simulink model "alignment_bending_procedure_n_4"  (R2018b)
settings: Solver=VariableStepAuto  StartTime=0.0  StopTime=3  RelTol=1e-3
values from neighbouring files (symbols this model uses):
  base_size = [0.2 0.3 1.5]    [robot_setup.m]    (also in robot_setup_bis.m)
  beam_length = 1.14    [robot_setup.m]    (also in robot_setup_bis.m)
  beam_radius = 0.032    [robot_setup.m]    (also in robot_setup_bis.m)
  beam_state_wf_des = fixture_keypoints(fixture_height, fixture_y, n_keypoints)    [robot_setup.m]    (also in robot_setup_bis.m)
  fixture_height = 1.5    [robot_setup.m]    (also in robot_setup_bis.m)
  fixture_x = 0.8    [robot_setup.m]    (also in robot_setup_bis.m)
  J = fscanf(fileID, '    [jacobian_mean_std.m]    (also in robot_setup.m = J_array{i-n_start+1}; robot_setup_bis.m = J_array{i-n_start+1})
  n_keypoints = i    [robot_setup.m]    (also in robot_setup_bis.m)
  robot_frame_x = 0.15    [robot_setup.m]    (also in robot_setup_bis.m)
  T = 0.005    [robot_setup.m]    (also in robot_setup_bis.m; sim_robot_control_error.m)
  wf_T_rf_left = [R_left, xyz_left'; 0 0 0 1]    [robot_setup.m]    (also in robot_setup_bis.m)
  wf_T_rf_right = [R_right, xyz_right'; 0 0 0 1]    [robot_setup.m]    (also in robot_setup_bis.m)
  xyz_0_rf_left = xyz_0_rf_left(1:3)    [robot_setup.m]    (also in robot_setup_bis.m)
  xyz_0_rf_right = xyz_0_rf_right(1:3)    [robot_setup.m]    (also in robot_setup_bis.m)
undefined symbols (not defined in the file or in its folder): beam_wall, beam_width, Extr_Data_Box, Levenberg, Marquardt, X, Y, Z
libraries: sm_lib x329, nesl_utility x49, sm_flex_body_lib x12, robotcorelib x4, simulink x2, robotmaniplib x2
(part 8 of 8)

== system alignment_bending_procedure_n_4/KUKA LWR right/KUKA_iiwa 1 /iiwa_link_7 ==
  Inertia : sm_lib/Body Elements/Inertia  InertiaType=Custom  Mass=3.129  MassUnits=kg  CenterOfMass=[0, 0, 0]  CenterOfMassUnits=m  MomentsOfInertia=[0.01464, 0.01465, 0.002872]  MomentsOfInertiaUnits=kg*m^2  ProductsOfInertia=[0, 0, 0.0005912]  ProductsOfInertiaUnits=kg*m^2  GraphicType=None  MarkerShape=Inertia  MarkerSize=20  GraphicVisPropType=SimpleVisualProperties  GraphicDiffuseColor=[0.5 0.5 0.5]  GraphicSpecularColor=[0.5 0.5 0.5 1.0]  GraphicAmbientColor=[0.15 0.15 0.15 1.0]  GraphicEmissiveColor=[0.0 0.0 0.0 1.0]  GraphicShininess=75  GraphicOpacity=1.0
  InertiaOriginTransform : sm_lib/Frames and Transforms/Rigid Transform  TranslationMethod=Cartesian  TranslationStandardOffset=0  TranslationLengthUnit=m  TranslationStandardAxis=+Z  TranslationCartesianOffset=[0, 0, 0.02]  TranslationROffset=0  TranslationROffsetUnits=m  TranslationZOffset=0  TranslationZOffsetUnits=m  TranslationThetaOffset=0  TranslationThetaOffsetUnits=deg  RotationMethod=RotationSequence  RotationAngleUnits=deg  RotationStandardAxis=+Z  RotationAngle=0.0  RotationArbitraryAxis=[0 0 1]  FollAlignAxisA=+X  BaseAlignAxisA=+Y  FollAlignAxisB=+Y  BaseAlignAxisB=+Z  RotationSequenceAxes=BaseAxes  RotationSequence=XYZ  RotationSequenceAngles=[0, 0, 0]  RotationSequenceAnglesUnits=rad  RotationMatrix=[1 0 0; 0 1 0; 0 0 1]
  ReferenceFrame : sm_lib/Frames and Transforms/Reference Frame
  Visual : sm_lib/Body Elements/Solid  InertiaType=Custom  Mass=0  MassUnits=kg  CenterOfMass=[0, 0, 0]  CenterOfMassUnits=m  MomentsOfInertia=[0, 0, 0]  MomentsOfInertiaUnits=kg*m^2  ProductsOfInertia=[0, 0, 0]  ProductsOfInertiaUnits=kg*m^2  BasedOnType=Density  Density=1000  DensityUnits=kg/m^3  DoExposeReferenceFrame=on  SerializedFrames=<Frames/>  GraphicType=FromGeometry  MarkerShape=Sphere  MarkerSize=10  GraphicVisPropType=SimpleVisualProperties  GraphicDiffuseColor=[0.4, 0.4, 0.4]  GraphicSpecularColor=[0.5 0.5 0.5 1.0]  GraphicAmbientColor=[0.15 0.15 0.15 1.0]  GraphicEmissiveColor=[0.0 0.0 0.0 1.0]  GraphicShininess=75  GraphicOpacity=1  GeometryShape=FromFile  RectangleSize=[1 1]  RectangleSizeUnits=m  BrickDimensions=[1 1 1]  BrickDimensionUnits=m  CylinderRadius=1  CylinderRadiusUnits=m  CylinderLength=1  CylinderLengthUnits=m  SphereRadius=1  SphereRadiusUnits=m  EllipsoidRadii=[1 1 1]  EllipsoidRadiiUnits=m  ExtrusionCrossSection=[1 1; -1 1; -1 -1; 1 -1]  ExtrusionCrossSectionUnits=m  ExtrusionLength=1  ExtrusionLengthUnits=m  PolygonNumSides=3  PolygonOuterRadius=1  PolygonOuterRadiusUnits=m  ExtGeomFileType=STL  ExtGeomFileName=iiwa_description/meshes/iiwa7/visual/link_7.stl  ExtGeomFileUnits=m  RevolutionCrossSection=[1 1; 1 -1; 2 -1; 2 1]  RevolutionCrossSectionUnits=m  RevolutionExtent=Full  RevolutionAngle=180  RevolutionAngleUnits=deg
  VisualOriginTransform : sm_lib/Frames and Transforms/Rigid Transform  TranslationMethod=Cartesian  TranslationStandardOffset=0  TranslationLengthUnit=m  TranslationStandardAxis=+Z  TranslationCartesianOffset=[0, 0, -0.0005]  TranslationROffset=0  TranslationROffsetUnits=m  TranslationZOffset=0  TranslationZOffsetUnits=m  TranslationThetaOffset=0  TranslationThetaOffsetUnits=deg  RotationMethod=RotationSequence  RotationAngleUnits=deg  RotationStandardAxis=+Z  RotationAngle=0.0  RotationArbitraryAxis=[0 0 1]  FollAlignAxisA=+X  BaseAlignAxisA=+Y  FollAlignAxisB=+Y  BaseAlignAxisB=+Z  RotationSequenceAxes=BaseAxes  RotationSequence=XYZ  RotationSequenceAngles=[0, 0, 0]  RotationSequenceAnglesUnits=rad  RotationMatrix=[1 0 0; 0 1 0; 0 0 1]
  iiwa_joint_7_AxisInvTransform : sm_lib/Frames and Transforms/Rigid Transform  TranslationMethod=Cartesian  TranslationStandardOffset=0  TranslationLengthUnit=m  TranslationStandardAxis=+Z  TranslationCartesianOffset=[0, 0, 0]  TranslationROffset=0  TranslationROffsetUnits=m  TranslationZOffset=0  TranslationZOffsetUnits=m  TranslationThetaOffset=0  TranslationThetaOffsetUnits=deg  RotationMethod=ArbitraryAxis  RotationAngleUnits=rad  RotationStandardAxis=+Z  RotationAngle=0  RotationArbitraryAxis=[1, 0, 0]  FollAlignAxisA=+X  BaseAlignAxisA=+Y  FollAlignAxisB=+Y  BaseAlignAxisB=+Z  RotationSequenceAxes=FollowerAxes  RotationSequence=XYX  RotationSequenceAngles=[0 0 0]  RotationSequenceAnglesUnits=deg  RotationMatrix=[1 0 0; 0 1 0; 0 0 1]
  iiwa_joint_ee_OriginTransform : sm_lib/Frames and Transforms/Rigid Transform  TranslationMethod=Cartesian  TranslationStandardOffset=0  TranslationLengthUnit=m  TranslationStandardAxis=+Z  TranslationCartesianOffset=[0, 0, 0.045]  TranslationROffset=0  TranslationROffsetUnits=m  TranslationZOffset=0  TranslationZOffsetUnits=m  TranslationThetaOffset=0  TranslationThetaOffsetUnits=deg  RotationMethod=RotationSequence  RotationAngleUnits=deg  RotationStandardAxis=+Z  RotationAngle=0.0  RotationArbitraryAxis=[0 0 1]  FollAlignAxisA=+X  BaseAlignAxisA=+Y  FollAlignAxisB=+Y  BaseAlignAxisB=+Z  RotationSequenceAxes=BaseAxes  RotationSequence=XYZ  RotationSequenceAngles=[0, -1.57079632679, 0]  RotationSequenceAnglesUnits=rad  RotationMatrix=[1 0 0; 0 1 0; 0 0 1]
  iiwa_joint_ee_kuka_OriginTransform : sm_lib/Frames and Transforms/Rigid Transform  TranslationMethod=Cartesian  TranslationStandardOffset=0  TranslationLengthUnit=m  TranslationStandardAxis=+Z  TranslationCartesianOffset=[0, 0, 0.045]  TranslationROffset=0  TranslationROffsetUnits=m  TranslationZOffset=0  TranslationZOffsetUnits=m  TranslationThetaOffset=0  TranslationThetaOffsetUnits=deg  RotationMethod=RotationSequence  RotationAngleUnits=deg  RotationStandardAxis=+Z  RotationAngle=0.0  RotationArbitraryAxis=[0 0 1]  FollAlignAxisA=+X  BaseAlignAxisA=+Y  FollAlignAxisB=+Y  BaseAlignAxisB=+Z  RotationSequenceAxes=BaseAxes  RotationSequence=XYZ  RotationSequenceAngles=[3.14159265359, 3.14159265359, 3.14159265359]  RotationSequenceAnglesUnits=rad  RotationMatrix=[1 0 0; 0 1 0; 0 0 1]
  F : PMIOPort  Side=Left
  F2 : PMIOPort  Port=2  Side=Right
  F1 : PMIOPort  Port=3  Side=Right
  connections:
  Inertia/RConn1 -- InertiaOriginTransform/RConn1
  ReferenceFrame/RConn1 -- InertiaOriginTransform/LConn1 -- iiwa_joint_ee_OriginTransform/LConn1 -- iiwa_joint_ee_kuka_OriginTransform/LConn1 -- iiwa_joint_7_AxisInvTransform/LConn1 -- VisualOriginTransform/LConn1
  Visual/RConn1 -- VisualOriginTransform/RConn1
  iiwa_joint_7_AxisInvTransform/RConn1 -- F/RConn1
  iiwa_joint_ee_OriginTransform/RConn1 -- F1/RConn1
  iiwa_joint_ee_kuka_OriginTransform/RConn1 -- F2/RConn1

== system alignment_bending_procedure_n_4/KUKA LWR right/KUKA_iiwa 1 /iiwa_link_ee_weld ==
  ReferenceFrame : sm_lib/Frames and Transforms/Reference Frame
  F : PMIOPort  Side=Left
  connections:
  ReferenceFrame/RConn1 -- F/RConn1

== system alignment_bending_procedure_n_4/KUKA LWR right/KUKA_iiwa 1 /world ==
  ReferenceFrame : sm_lib/Frames and Transforms/Reference Frame
  world_iiwa_joint_OriginTransform : sm_lib/Frames and Transforms/Rigid Transform  TranslationMethod=Cartesian  TranslationStandardOffset=0  TranslationLengthUnit=m  TranslationStandardAxis=+Z  TranslationCartesianOffset=base_pos  TranslationROffset=0  TranslationROffsetUnits=m  TranslationZOffset=0  TranslationZOffsetUnits=m  TranslationThetaOffset=0  TranslationThetaOffsetUnits=deg  RotationMethod=RotationSequence  RotationAngleUnits=deg  RotationStandardAxis=+Z  RotationAngle=0.0  RotationArbitraryAxis=[0 0 1]  FollAlignAxisA=+X  BaseAlignAxisA=+Y  FollAlignAxisB=+Y  BaseAlignAxisB=+Z  RotationSequenceAxes=BaseAxes  RotationSequence=ZYX  RotationSequenceAngles=base_rot  RotationSequenceAnglesUnits=rad  RotationMatrix=[1 0 0; 0 1 0; 0 0 1]
  F : PMIOPort  Side=Left
  F1 : PMIOPort  Port=2  Side=Right
  connections:
  world_iiwa_joint_OriginTransform/LConn1 -- ReferenceFrame/RConn1 -- F/RConn1
  world_iiwa_joint_OriginTransform/RConn1 -- F1/RConn1

== matlab function alignment_bending_procedure_n_4/Subsystem/deformation ctrl ==
  data: beam_state_wf input; beam_state_wf_des input; deformation_state_des_new output; J input; x_wf_des input; deformation_state input; deformation_state_des_old input; n_iterations_old input; n_iterations_new output
%idea, after the arrive of measurements from beam and end-effectors


function [deformation_state_des_new, n_iterations_new] = deformation_ctrl(beam_state_wf, beam_state_wf_des, J,  x_wf_des, deformation_state, deformation_state_des_old, n_iterations_old)

    thresh_deformation = 0.001;
    thresh_beam_state_err = 0.01;

    n_iterations_des = 1;
    n_iterations_new=n_iterations_old;

    %compute alignment error
    err=beam_state_wf_des-beam_state_wf;
    deformation_state_des_new = deformation_state_des_old;
    
    
    if norm(beam_state_wf)< 10 %&& (n_iterations_new < n_iterations_des) 
        
        n_iterations_new=n_iterations_old+1;
        n_states = length(deformation_state);
        deformation_state_des_new(1:n_states-1) = deformation_state(1:n_states-1)+pinv(J)*err;
        
        deformation_state_des_new(n_states) = 0.8*x_wf_des;
        
    end

    %cond = norm(beam_state_wf) > 10 || ...
    %    norm(err) < thresh_beam_state_err || ...
    %    norm(deformation_state_des_new-deformation_state) < thresh_deformation || ... 
    %    n_iterations_old >= n_iterations_des;

    %if ~cond
        %H = J'*J;
        %f = -err'*J;
        %deformation_state_des = quadprog(H,f);
        
    %end

end

== matlab function alignment_bending_procedure_n_4/CONTROLLER1/CONTROLLER/Controller ==
  data: T input; yz_beam_wf input; xyz_beam_wf_des input; xyz_rf_new output; wf_T_rf_left input; wf_T_rf_right input; ypr_rf_old input; xyz_rf_old input; trigger_old input; ypr_rf_new output; trigger_new output; iterations_old input; iterations_new output
function [ xyz_rf_new, ypr_rf_new, trigger_new, iterations_new]   = robot_ctrl(T, yz_beam_wf, xyz_beam_wf_des, wf_T_rf_left, wf_T_rf_right, ypr_rf_old, xyz_rf_old, trigger_old, iterations_old)  

    thresh_l = 10^-3;
    
    lambda = 2;
    if(iterations_old<0.05/T)
        lambda = 0;
    end
    iterations_new = iterations_old+1;
    
    
    trigger_new = trigger_old;
    
    ypr_rf_new_left = ypr_rf_old(1:3);
    ypr_rf_new_right = ypr_rf_old(4:6);
   
    xyz_rf_new_left = xyz_rf_old(1:3);
    xyz_rf_new_right = xyz_rf_old(4:6);
    
     % work in the world frame
    xyz_wf_new_left = wf_T_rf_left * [xyz_rf_new_left;1];
    xyz_wf_new_right = wf_T_rf_right * [xyz_rf_new_right;1];    

    yd_wf_des = xyz_beam_wf_des(1);
    ym_wf_des = xyz_beam_wf_des(2);
    zd_wf_des = xyz_beam_wf_des(3);
    zm_wf_des = xyz_beam_wf_des(4);
    xm_wf_des = xyz_beam_wf_des(end);
    
    x_wf_new_left = xyz_wf_new_left(1);
    x_wf_new_right = xyz_wf_new_right(1);
    y_wf_new_left = xyz_wf_new_left(2);
    y_wf_new_right = xyz_wf_new_right(2);
    z_wf_new_left = xyz_wf_new_left(3);
    z_wf_new_right = xyz_wf_new_right(3);
    
    yd_wf = y_wf_new_left-y_wf_new_right;
    ym_wf = (y_wf_new_left+y_wf_new_right)/2;
    zd_wf = z_wf_new_left-z_wf_new_right;
    zm_wf = (z_wf_new_left+z_wf_new_right)/2;
    xm_wf = (x_wf_new_left+x_wf_new_right)/2;
    
    cond_yd = abs(yd_wf_des-yd_wf) < thresh_l;  
    cond_ym = abs(ym_wf_des-ym_wf) < thresh_l;
    cond_zd = abs(zd_wf_des-zd_wf) < thresh_l;
    cond_zm = abs(zm_wf_des-zm_wf) < thresh_l;
    cond_xm = abs(xm_wf_des-xm_wf) < thresh_l;
    
    %% relative distance along y (wf)
    if cond_yd
        trigger_new(1,1) = 1;
    end

    %% absolute distance from origin
    if cond_ym 
        trigger_new(2,1) = 1;
    end
    
    %% relative distance along z (wf)
    if cond_zd
        trigger_new(3,1) = 1;
    end 
    
    %% absolute distance along z (wf)
    if cond_zm
        trigger_new(4,1) = 1;
    end 
    
    %% absolute distance along x (wf)
    if cond_xm
        trigger_new(5,1) = 1;
    end 
    
    % relative distance along y (wf)
    if ~cond_yd && trigger_new(1,1) == 0
  
        [xyz_wf_new_left(2), xyz_wf_new_right(2)] = symmetric_pos_ctrl(yd_wf, yd_wf_des, lambda, T, -1, xyz_wf_new_left(2), xyz_wf_new_right(2));
    
        % absolute distance along y (wf)
    elseif ~cond_ym && trigger_new(2,1)==0
              
        [xyz_wf_new_left(2), xyz_wf_new_right(2)] = symmetric_pos_ctrl(ym_wf, ym_wf_des, lambda, T, 1, xyz_wf_new_left(2), xyz_wf_new_right(2));
        
    % relative distance along z (wf)
    elseif ~cond_zd && trigger_new(3,1) == 0
  
        [xyz_wf_new_left(3), xyz_wf_new_right(3)] = symmetric_pos_ctrl(zd_wf, zd_wf_des, 0.5*lambda, T, -1, xyz_wf_new_left(3), xyz_wf_new_right(3));
    
    % absolute distance along z (wf)
    elseif ~cond_zm && trigger_new(4,1) == 0
  
        [xyz_wf_new_left(3), xyz_wf_new_right(3)] = symmetric_pos_ctrl(zm_wf, zm_wf_des, lambda, T, 1, xyz_wf_new_left(3), xyz_wf_new_right(3));
    
     % absolute distance along x (wf)
     elseif ~cond_xm && trigger_new(5,1) == 0

        [xyz_wf_new_left(1), xyz_wf_new_right(1)] = symmetric_pos_ctrl(xm_wf, xm_wf_des, lambda, T, 1, xyz_wf_new_left(1), xyz_wf_new_right(1));

    end
    
    xyz_rf_new_left = (wf_T_rf_left^-1)*xyz_wf_new_left;
    xyz_rf_new_right = (wf_T_rf_right^-1)*xyz_wf_new_right;
    
    ypr_rf_new = [ypr_rf_new_left;ypr_rf_new_right];
    xyz_rf_new = [xyz_rf_new_left(1:3);xyz_rf_new_right(1:3)];
    
    
    
    

end

== matlab function alignment_bending_procedure_n_4/Subsystem/deformation_input_msr ==
  data: xyz_rf_left input; deformation_state output; xyz_rf_right input; wf_T_rf_left input; wf_T_rf_right input
function deformation_state = deformation_input_msr(xyz_rf_left, xyz_rf_right, wf_T_rf_left, wf_T_rf_right)

    xyz_wf_left=wf_T_rf_left*[xyz_rf_left;1];
    xyz_wf_right=wf_T_rf_right*[xyz_rf_right;1];

    x_wf_left = xyz_wf_left(1);
    x_wf_right = xyz_wf_right(1);
    y_wf_left = xyz_wf_left(2);
    y_wf_right = xyz_wf_right(2);
    z_wf_left = xyz_wf_left(3);
    z_wf_right = xyz_wf_right(3);
    
    yd_wf = y_wf_left-y_wf_right;
    ym_wf = (y_wf_left+y_wf_right)/2;
    zd_wf = z_wf_left-z_wf_right;
    zm_wf = (z_wf_left+z_wf_right)/2;
    xm_wf = (x_wf_left+x_wf_right)/2;
    
    deformation_state = [yd_wf, ym_wf, zd_wf, zm_wf, xm_wf]';
 
end

== matlab function alignment_bending_procedure_n_4/BEAM1/MATLAB Function1 ==
  data: u input; y output; n_keypoints input
function y = error_measure(u, n_keypoints)

    y = norm(u)/n_keypoints;
end
